simulink model "Identification_Simscape"  (R2015a)
settings: Solver=ode23t  StartTime=0.0  StopTime=10.0  FixedStep=-0.01  RelTol=1e-3
InitFcn:
  | load('LeftInput_Measures.mat');
  | load('LeftOutput_Measures.mat');
  | Parametres_Rover
libraries: SingleMotor_Duty_to_inc x2, SingleMotor_V_to_rads x1
settings Model: Creator=tbaroche  LastModifiedBy=tbaroche

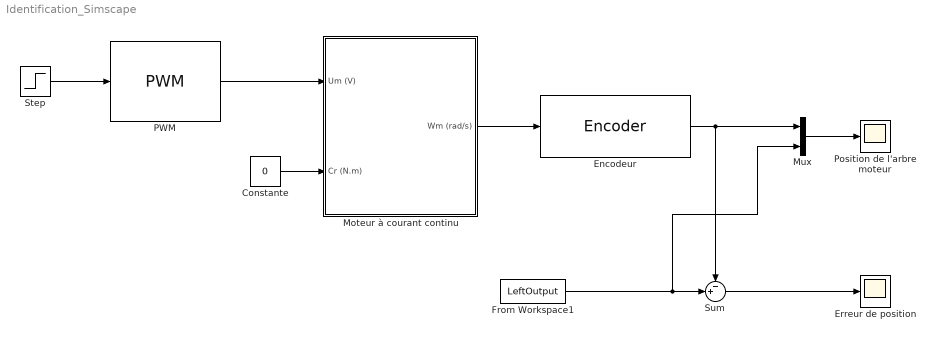
== system Identification_Simscape ==
  Constante : Constant  Value=0
  Encodeur : SingleMotor_Duty_to_inc/Encoder  EncRes=EncRes
  Erreur de position : Scope
      settings: TimeRange=10  YMin=-1300  YMax=100
  From Workspace1 : FromWorkspace  VariableName=LeftOutput  SampleTime=0
  Moteur à courant continu : Subsystem  BlockChoice=Modèle Simscape
      link override "SimElectronics Model ": Kphi_lib=Kphi  Rm_lib=Rm  Lm_lib=Lm  bm_lib=bm  Jm_lib=Jm
      settings: AttributesFormatString=%<BlockChoice>  TemplateBlock=SingleMotor_V_to_rads/DC Motor  MemberBlocks=Modèle Simscape,Modèle Simulink
  Mux : Mux  Inputs=2
  PWM : SingleMotor_Duty_to_inc/PWM  FreqTriangle=FreqPWM
  Position de l'arbre moteur : Scope
      settings: YMin=0  YMax=8500
  Step : Step  Time=3  After=50  SampleTime=0
  Sum : Sum  Inputs=-+|
  wires:
  Moteur à courant continu/1(Wm (rad/s)) -> Encodeur/1
  Step/1 -> PWM/1
  From Workspace1/1 -> Mux/2, Sum/2
  Sum/1 -> Erreur de position/1
  Encodeur/1 -> Mux/1, Sum/1
  Mux/1 -> Position de l'arbre moteur/1
  Constante/1 -> Moteur à courant continu/2(Cr (N.m))
  PWM/1 -> Moteur à courant continu/1(Um (V))

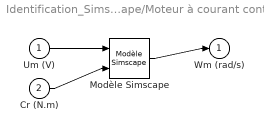
== system Identification_Simscape/Moteur à courant continu ==
  Um (V) : Inport
  Cr (N.m) : Inport  Port=2
  Modèle Simscape : SingleMotor_V_to_rads/Modèle Simscape  Kphi_lib=Kphi  Rm_lib=Rm  Lm_lib=Lm  bm_lib=bm  Jm_lib=Jm
  Wm (rad/s) : Outport
  wires:
  Um (V)/1 -> Modèle Simscape/1
  Cr (N.m)/1 -> Modèle Simscape/2
  Modèle Simscape/1 -> Wm (rad/s)/1
